simulink model "verify_Simple_House_ISOgm_CONF_mdl"  (R2016b)
settings: Solver=ode45  StartTime=0  StopTime=365*24*3600  RelTol=1e-3  EnableMultiTasking=on
InitFcn:
  | load('DE_TRY2010_04_averageYear')
undefined symbols (not defined in the file or in its folder): path_carnot
libraries: carnot x3
settings Model: Creator=drhf  LastModifiedBy=drhf
settings DataIOCC: SaveFormat=Array  SignalLoggingSaveFormat=ModelDataLogs
settings OptimizationCC: ExpressionDepthLimit=2147483647  LifeSpan=inf
settings DebuggingCC: UnderspecifiedInitializationDetection=Classic  MergeDetectMultiDrivingBlocksExec=none  SolverPrmCheckMsg=warning  FcnCallInpInsideContextMsg=warning  StateNameClashWarn=warning  SFUnexpectedBacktrackingDiag=warning  SFNoUnconditionalDefaultTransitionDiag=warning  SFExecutionAtInitializationDiag=none
settings HardwareCC: ProdBitPerPointer=32  ProdBitPerSizeT=32  ProdBitPerPtrDiffT=32  ProdLargestAtomicFloat=None  ProdIntDivRoundTo=Undefined  ProdEndianess=Unspecified  ProdWordSize=32  ProdHWDeviceType=32-bit Generic
settings ModelReferenceCC: PropagateSignalLabelsOutOfModel=off
settings GRTTargetCC: TargetLangStandard=C89/C90 (ANSI)  GeneratePreprocessorConditionals=Disable all  CombineOutputUpdateFcns=off  GRTInterface=on
settings ConfigComp: CovMetricSettings=dw  CovHtmlReporting=on  CovSaveCumulativeToWorkspaceVar=on  CovSaveSingleToWorkspaceVar=on  CovExternalEMLEnable=off

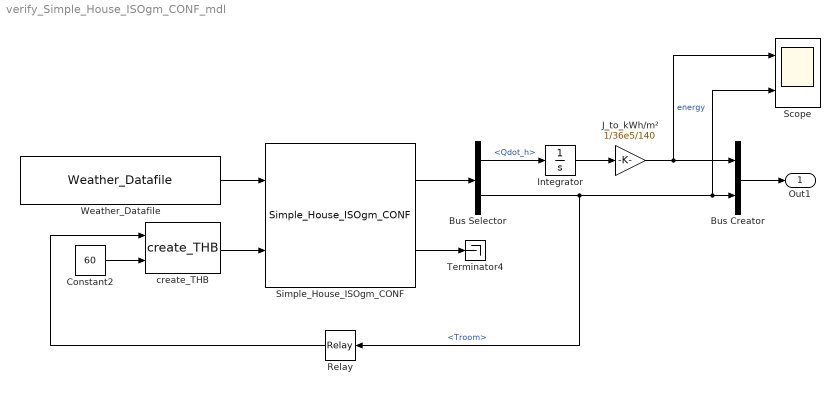
== system verify_Simple_House_ISOgm_CONF_mdl ==
  Bus Creator : BusCreator  Inputs=2
  Bus Selector : BusSelector  OutputSignals=Qdot.Qdot_h,Troom
  Constant2 : Constant  Value=60
  Integrator : Integrator
  J_to_kWh/m² : Gain  Gain=1/36e5/140
  Relay : Relay  OnSwitchValue=20.1  OffSwitchValue=19.9  OnOutputValue=0  OffOutputValue=800/3600
  Scope : Scope  NumInputPorts=2
  Simple_House_ISOgm_CONF : carnot/Load/Houses/Simple_House_ISOgm_CONF  tini=20  PathName=fullfile(path_carnot('libsl'),'Load','Houses','Simple_House_ISOgm_CONF','parameter_set')  FileName='Default_SimpleHouseISOgm.mat'  userPath=off  userParam=off  Ahabit=140  Hroom=2.5  Slab=[7 10]  UAwall=100  UAneighbour=0  Uground=0.7  cap=70000000  Awindow=[12 4 3 4]  AziWindow=[0 90 -180 -90]  Uwindow=[2 2 2 2]  Gwindow=[0.5 0.5 0.5 0.5]  shading=0.75  Ventilationrate=0.4  Heatrecovery=0  Heatload=4500  DTnomHeatingsystem=15  RadiatorExponent=1.1  CapHeatingsystem=40000000  DpHeatingsystem=[10 10]
  Terminator4 : Terminator
  Weather_Datafile : carnot/Weather/Weather_Datafile  PathName='C:\repos\carnot_svn\trunk\public\data\'  FileName='DE_TRY2010_04_averageYear.mat'  UserParam=off  VariableName=DE_TRY2010_04_averageYear  SampleTime=3600
  create_THB : carnot/Source/Simple/create_THB  p=1e5  fluid=Water  mix=0  mix2=0  mix3=0  dia=0.02  hgt=0  mID=No Pressure Drop
  Out1 : Outport
  wires:
  Weather_Datafile/1 -> Simple_House_ISOgm_CONF/1
  Bus Creator/1 -> Out1/1
  Simple_House_ISOgm_CONF/2 -> Terminator4/1
  Simple_House_ISOgm_CONF/1 -> Bus Selector/1
  Bus Selector/2 -> Relay/1, Bus Creator/2, Scope/2  "<Troom>"
  Constant2/1 -> create_THB/2
  Relay/1 -> create_THB/1
  create_THB/1 -> Simple_House_ISOgm_CONF/2
  Bus Selector/1 -> Integrator/1  "<Qdot_h>"
  Integrator/1 -> J_to_kWh/m²/1
  J_to_kWh/m²/1 -> Scope/1, Bus Creator/1  "energy"
